simulink model "Desorbtion_mt_2"  (R2018b)
settings: Solver=ode3  StartTime=0.0  StopTime=1000000  FixedStep=0.1  RelTol=1e-3  EnableMultiTasking=on
settings Model: Creator=User  LastModifiedBy=user
settings DataIOCC: LimitDataPoints=on  SaveFormat=Array  SignalLoggingSaveFormat=ModelDataLogs
settings OptimizationCC: ExpressionDepthLimit=2147483647  InitFltsAndDblsToZero=on  LifeSpan=inf
settings DebuggingCC: UnderspecifiedInitializationDetection=Classic  MergeDetectMultiDrivingBlocksExec=none  SolverPrmCheckMsg=warning  FcnCallInpInsideContextMsg=warning  StateNameClashWarn=warning  SFUnexpectedBacktrackingDiag=warning  SFNoUnconditionalDefaultTransitionDiag=warning  SFExecutionAtInitializationDiag=none
settings HardwareCC: ProdBitPerPointer=32  ProdBitPerSizeT=32  ProdBitPerPtrDiffT=32  ProdLargestAtomicFloat=None  ProdIntDivRoundTo=Undefined  ProdEndianess=Unspecified  ProdWordSize=32  ProdHWDeviceType=32-bit Generic
settings ModelReferenceCC: PropagateSignalLabelsOutOfModel=off
settings SFSimCC: SimUseLocalCustomCode=off
settings RTWCC: RTWUseLocalCustomCode=off
settings CodeAppCC: StateflowObjectComments=on
settings GRTTargetCC: TargetLangStandard=C89/C90 (ANSI)  GeneratePreprocessorConditionals=Disable all  CombineOutputUpdateFcns=off  GRTInterface=on
settings ConfigComp: CovMetricSettings=dw  CovHtmlReporting=on  CovSaveCumulativeToWorkspaceVar=on  CovSaveSingleToWorkspaceVar=on  CovExternalEMLEnable=off  CovSFcnEnable=off

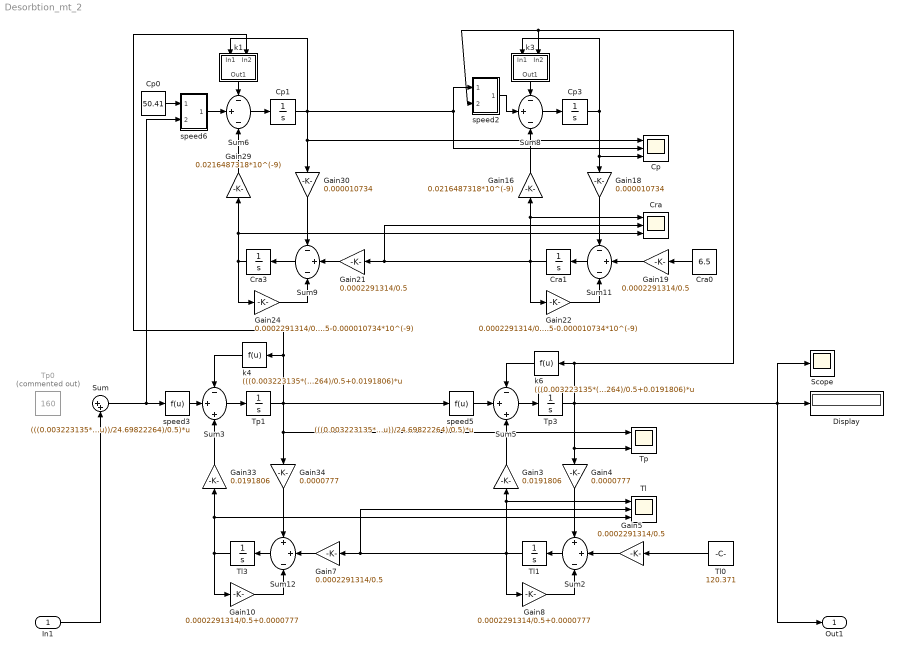
== system Desorbtion_mt_2 ==
  In1 : Inport
  Cp : Scope  NumInputPorts=3
  Cp0 : Constant  Value=50.41
  Cp1 : Integrator  InitialCondition=62.8910352690798
  Cp3 : Integrator  InitialCondition=97.0647284967471
  Cra : Scope  NumInputPorts=3
  Cra0 : Constant  Value=6.5
  Cra1 : Integrator  InitialCondition=4.2264294731348
  Cra3 : Integrator  InitialCondition=0.9249430199510
  Display : Display
  Gain10 : Gain  Gain=0.0002291314/0.5+0.0000777
  Gain16 : Gain  Gain=0.0216487318*10^(-9)
  Gain18 : Gain  Gain=0.000010734
  Gain{5,7,19,21} (4 alike) : Gain  Gain=0.0002291314/0.5
  Gain22 : Gain  Gain=0.0002291314/0.5-0.000010734*10^(-9)
  Gain24 : Gain  Gain=0.0002291314/0.5-0.000010734*10^(-9)
  Gain29 : Gain  Gain=0.0216487318*10^(-9)
  Gain3 : Gain  Gain=0.0191806
  Gain30 : Gain  Gain=0.000010734
  Gain33 : Gain  Gain=0.0191806
  Gain34 : Gain  Gain=0.0000777
  Gain4 : Gain  Gain=0.0000777
  Gain8 : Gain  Gain=0.0002291314/0.5+0.0000777
  Scope : Scope
  Sum : Sum  Inputs=|++
  Sum{6,8..9,11} (4 alike) : Sum  Inputs=-+-
  Sum12 : Sum  Inputs=++-
  Sum2 : Sum  Inputs=++-
  Sum3 : Sum  Inputs=-++
  Sum5 : Sum  Inputs=-++
  Tl : Scope  NumInputPorts=3
  Tl0 : Constant  Value=120.371
  Tl1 : Integrator  InitialCondition=124.7521008288133
  Tl3 : Integrator  InitialCondition=133.0396819538713
  Tp : Scope  NumInputPorts=3
  Tp0 : Constant  Commented=on  Value=160
  Tp1 : Integrator  InitialCondition=157.0139168404367
  Tp3 : Integrator  InitialCondition=150.5911681762652  IgnoreLimit=on
  k1 : Subsystem
  k3 : Subsystem
  k4 : Fcn  Expr=(((0.003223135*(273+u))/24.69822264)/0.5+0.0191806)*u
  k6 : Fcn  Expr=(((0.003223135*(273+u))/24.69822264)/0.5+0.0191806)*u
  speed2 : Subsystem
  speed3 : Fcn  Expr=(((0.003223135*(273+u))/24.69822264)/0.5)*u
  speed5 : Fcn  Expr=(((0.003223135*(273+u))/24.69822264)/0.5)*u
  speed6 : Subsystem
  Out1 : Outport
  wires:
  Sum6/1 -> Cp1/1
  speed2/1(Out1) -> Sum8/2
  Sum8/1 -> Cp3/1
  Cp1/1 -> Cp/2, speed2/1(In1), Gain30/1, Cp/1, k1/1(In1)
  Gain29/1 -> Sum6/3
  Cp3/1 -> Gain18/1, Cp/3, k3/1(In1)
  Gain16/1 -> Sum8/3
  Gain30/1 -> Sum9/1
  Gain18/1 -> Sum11/1
  Gain19/1 -> Sum11/2
  Sum11/1 -> Cra1/1
  Cra1/1 -> Gain21/1, Cra/2, Gain22/1, Gain16/1, Cra/1
  Gain21/1 -> Sum9/2
  Sum9/1 -> Cra3/1
  Cra3/1 -> Gain24/1, Gain29/1, Cra/3
  Gain22/1 -> Sum11/3
  Gain24/1 -> Sum9/3
  speed3/1 -> Sum3/2
  k4/1 -> Sum3/1
  Sum3/1 -> Tp1/1
  speed5/1 -> Sum5/2
  k6/1 -> Sum5/1
  Sum5/1 -> Tp3/1
  Tp1/1 -> speed5/1, Gain34/1, Tp/1, k4/1, k1/2(In2)
  Gain33/1 -> Sum3/3
  Tp3/1 -> Gain4/1, Tp/3, Out1/1, Scope/1, Display/1, k6/1, k3/2(In2), speed2/2(In2)
  Gain3/1 -> Sum5/3
  Gain34/1 -> Sum12/1
  Gain4/1 -> Sum2/1
  Gain5/1 -> Sum2/2
  Sum2/1 -> Tl1/1
  Tl1/1 -> Gain7/1, Tl/2, Gain8/1, Gain3/1, Tl/1
  Gain7/1 -> Sum12/2
  Sum12/1 -> Tl3/1
  Tl3/1 -> Gain10/1, Gain33/1, Tl/3
  Gain8/1 -> Sum2/3
  Gain10/1 -> Sum12/3
  speed6/1(Out1) -> Sum6/2
  Cp0/1 -> speed6/1(In1)
  k1/1(Out1) -> Sum6/1
  k3/1(Out1) -> Sum8/1
  Cra0/1 -> Gain19/1
  Sum/1 -> speed6/2(In2), speed3/1
  Tl0/1 -> Gain5/1
  In1/1 -> Sum/2

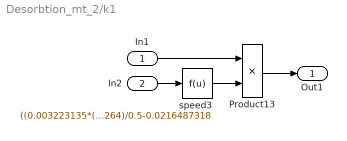
== system Desorbtion_mt_2/k1 ==
  In1 : Inport
  In2 : Inport  Port=2
  Product13 : Product  SaturateOnIntegerOverflow=on  InputSameDT=on  OutDataTypeStr=Inherit: Same as first input
  speed3 : Fcn  Expr=((0.003223135*(273+u))/24.69822264)/0.5-0.0216487318
  Out1 : Outport
  wires:
  Product13/1 -> Out1/1
  speed3/1 -> Product13/2
  In2/1 -> speed3/1
  In1/1 -> Product13/1

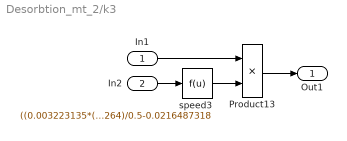
== system Desorbtion_mt_2/k3 ==
  In1 : Inport
  In2 : Inport  Port=2
  Product13 : Product  SaturateOnIntegerOverflow=on  InputSameDT=on  OutDataTypeStr=Inherit: Same as first input
  speed3 : Fcn  Expr=((0.003223135*(273+u))/24.69822264)/0.5-0.0216487318
  Out1 : Outport
  wires:
  Product13/1 -> Out1/1
  speed3/1 -> Product13/2
  In2/1 -> speed3/1
  In1/1 -> Product13/1

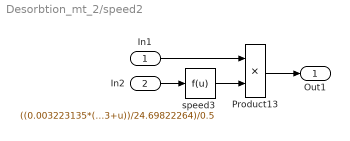
== system Desorbtion_mt_2/speed2 ==
  In1 : Inport
  In2 : Inport  Port=2
  Product13 : Product  SaturateOnIntegerOverflow=on  InputSameDT=on  OutDataTypeStr=Inherit: Same as first input
  speed3 : Fcn  Expr=((0.003223135*(273+u))/24.69822264)/0.5
  Out1 : Outport
  wires:
  In1/1 -> Product13/1
  In2/1 -> speed3/1
  speed3/1 -> Product13/2
  Product13/1 -> Out1/1

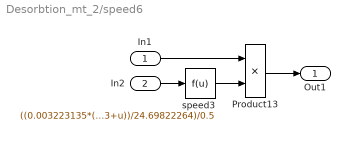
== system Desorbtion_mt_2/speed6 ==
  In1 : Inport
  In2 : Inport  Port=2
  Product13 : Product  SaturateOnIntegerOverflow=on  InputSameDT=on  OutDataTypeStr=Inherit: Same as first input
  speed3 : Fcn  Expr=((0.003223135*(273+u))/24.69822264)/0.5
  Out1 : Outport
  wires:
  In1/1 -> Product13/1
  In2/1 -> speed3/1
  speed3/1 -> Product13/2
  Product13/1 -> Out1/1
